simulink model "final_project"  (R2024b)
settings: Solver=FixedStepAuto  StartTime=0.0  StopTime=5  FixedStep=1e-6  RelTol=1e-3
model workspace (MAT data in the model file):
  Vdc = 1200
  fs = 15000
libraries: spsIGBTDiodeLib x6, spsGroundLib x3, simulink x3, spsMultimeterLib x2, spsSeriesRLCBranchLib x2, spsThreePhaseVIMeasurementLib x2, spsAsynchronousMachineSIUnitsLib x1, spsDCVoltageSourceLib x1, spsPower3phInstantaneousLib x1, spsThreePhaseParallelRLCBranchLib x1, spsThreePhaseSeriesRLCBranchLib x1, spsVoltageMeasurementLib x1
settings Model: Creator=zachary.newsom  LastModifiedBy=zachary.newsom

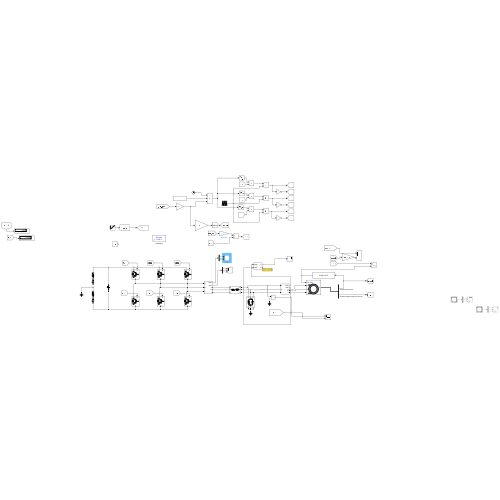
[thumbnail: Simulink's stored preview of the top-level diagram]
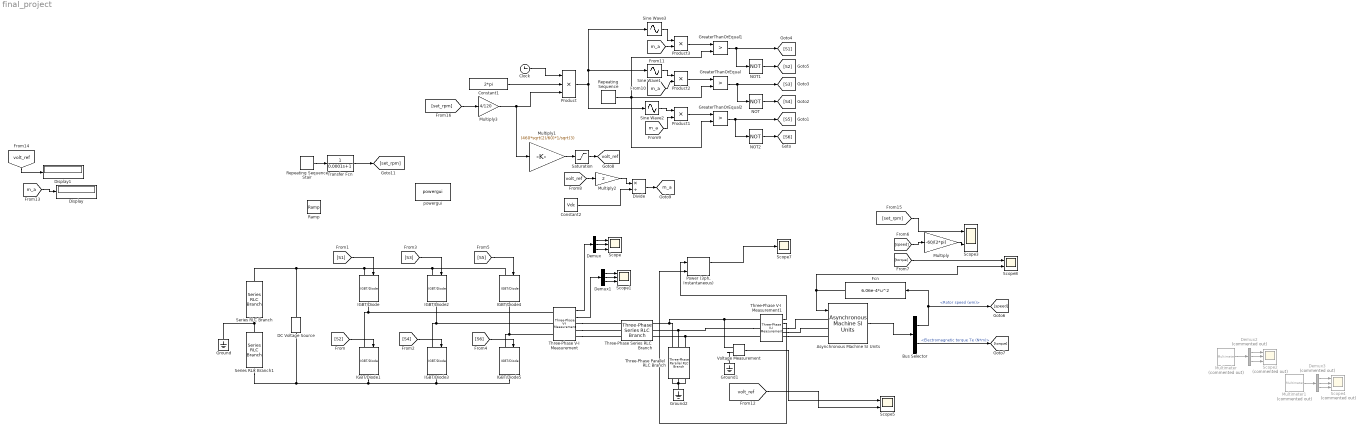
== system final_project ==
  Asynchronous Machine SI Units : spsAsynchronousMachineSIUnitsLib/Asynchronous Machine SI Units  RotorType=Squirrel-cage  PresetModel="01:  5 HP   460 V 60Hz 1750 RPM"  MechanicalLoad=Torque Tm  ShowDetailedParameters=on  ReferenceFrame=Rotor  Units=SI  MeasurementBus=off  NominalParameters=[3730 460 60]  VoltageRatio=1  Stator=[1.115 0.005974]  Rotor=[1.083 0.005974]  Cage1=[0.4155 0.002066]  Cage2=[0.4168 0.0003495]  Lm=0.2037  Mechanical=[0.02 0.005752 2]  PolePairs=2  InitialConditions=[1 0 0 0 0 0 0 0]  SimulateSaturation=off  Saturation=[14.03593122, 27.81365428, 53.79336849, 72.68890987, 97.98006896, 148.6815601, 215.7428561, 302.9841135, 428.7778367 ; 230, 322, 414, 460, 506, 552, 598, 644, 690]  LoadFlowParameters=1492000  TsPowergui=0  TsBlock=-1  IterativeModel=Trapezoidal non iterative  IterativeDiscreteModel=Trapezoidal robust  Pmec=1.492e+006
  Bus Selector : BusSelector  OutputSignals=Mechanical.Rotor speed (wm),Mechanical.Electromagnetic torque Te (N*m)
  Clock : Clock
  Constant1 : Constant  Value=2*pi
  Constant2 : Constant  Value=Vdc
  DC Voltage Source : spsDCVoltageSourceLib/DC Voltage Source  Amplitude=Vdc  Measurements=None
  Demux : Demux  Outputs=3
  Demux1 : Demux  Outputs=3
  Demux2 : Demux  Commented=on  Outputs=3
  Demux3 : Demux  Commented=on  Outputs=3
  Display : Display
  Display1 : Display
  Divide : Product  Inputs=*/
  Fcn : Fcn  Expr=6.06e-4*u^2
  GreaterThanOrEqual : RelationalOperator  Operator=>  OutDataTypeStr=boolean  RndMeth=Simplest  InputSameDT=off
  GreaterThanOrEqual1 : RelationalOperator  Operator=>  OutDataTypeStr=boolean  RndMeth=Simplest  InputSameDT=off
  GreaterThanOrEqual2 : RelationalOperator  Operator=>  OutDataTypeStr=boolean  RndMeth=Simplest  InputSameDT=off
  Ground : spsGroundLib/Ground  LConnTagsString=a
  Ground1 : spsGroundLib/Ground  LConnTagsString=a
  Ground2 : spsGroundLib/Ground  LConnTagsString=a
  IGBT/Diode{,1..3} (4 alike) : spsIGBTDiodeLib/IGBT//Diode  Ron=1e-6  Rs=1e5  Cs=inf  Measurements=off
  IGBT/Diode4 : spsIGBTDiodeLib/IGBT//Diode  Ron=1e-3  Rs=1e5  Cs=inf  Measurements=off
  IGBT/Diode5 : spsIGBTDiodeLib/IGBT//Diode  Ron=1e-3  Rs=1e5  Cs=inf  Measurements=off
  Multimeter : spsMultimeterLib/Multimeter  Commented=on  L=3  sel=1  yselected={}  Gain=0  OutputType=Complex  PlotAtSimulationStop=off  PhasorSimulation=off
  Multimeter1 : spsMultimeterLib/Multimeter  Commented=on  L=3  sel=1  yselected={}  Gain=0  OutputType=Complex  PlotAtSimulationStop=off  PhasorSimulation=off
  Multiply : Gain  Gain=-60/(2*pi)
  Multiply1 : Gain  Gain=(460*sqrt(2)/60)*1/sqrt(3)
  Multiply2 : Gain  Gain=2
  Multiply3 : Gain  Gain=4/120
  NOT : Logic  Operator=NOT  IconShape=distinctive  AllPortsSameDT=off  OutDataTypeStr=boolean
  NOT1 : Logic  Operator=NOT  IconShape=distinctive  AllPortsSameDT=off  OutDataTypeStr=boolean
  NOT2 : Logic  Operator=NOT  IconShape=distinctive  AllPortsSameDT=off  OutDataTypeStr=boolean
  "Power (3ph, Instantaneous)" : spsPower3phInstantaneousLib/Power (3ph, Instantaneous)
  Product : Product  Inputs=3
  Product1 : Product
  Product2 : Product
  Product3 : Product
  Ramp : simulink/Sources/Ramp  slope=1000  start=0  InitialOutput=400
  Repeating Sequence : simulink/Sources/Repeating Sequence  rep_seq_t=[0 0.5 1]/fs  rep_seq_y=[-1 1 -1]
  Repeating Sequence Stair : simulink/Sources/Repeating Sequence Stair  OutValues=[250 500 750 1000 1250 1500 1750].'  tsamp=0.5  OutMin=[]  OutMax=[]  OutDataTypeStr=double  OutputDataTypeScalingMode=double  OutDataType=fixdt(0,8)  ConRadixGroup=Best Precision: Vector-wise  OutScaling=2^-12
  Saturation : Saturate  UpperLimit=Vdc/2  LowerLimit=20
  Scope : Scope  NumInputPorts=3
  Scope1 : Scope  NumInputPorts=3
  Scope2 : Scope  Commented=on  NumInputPorts=3
  Scope3 : Scope  NumInputPorts=2
  Scope4 : Scope  Commented=on  NumInputPorts=3
  Scope5 : Scope  NumInputPorts=2
  Scope7 : Scope
  Scope8 : Scope  NumInputPorts=2
  Series RLC Branch : spsSeriesRLCBranchLib/Series RLC Branch  LConnTagsString=__new0  RConnTagsString=__new0  BranchType=RC  Resistance=1e6  Inductance=1e-3  SetiL0=off  InitialCurrent=0  Capacitance=1e-3  Setx0=off  InitialVoltage=0  Measurements=None
  Series RLC Branch1 : spsSeriesRLCBranchLib/Series RLC Branch  LConnTagsString=__new0  RConnTagsString=__new0  BranchType=RC  Resistance=1e6  Inductance=1e-3  SetiL0=off  InitialCurrent=0  Capacitance=1e-3  Setx0=off  InitialVoltage=0  Measurements=None
  Sine Wave1 : Sin  TimeSource=Use external signal  Phase=2*pi/3  SampleTime=0
  Sine Wave2 : Sin  TimeSource=Use external signal  Phase=4*pi/3  SampleTime=0
  Sine Wave3 : Sin  TimeSource=Use external signal  SampleTime=0
  Three-Phase Parallel RLC Branch : spsThreePhaseParallelRLCBranchLib/Three-Phase Parallel RLC Branch  LConnTagsString=A|B|C  RConnTagsString=A|B|C  BranchType=RC  Resistance=1e6  Inductance=1e-3  Capacitance=258e-6  Measurements=None
  Three-Phase Series RLC Branch : spsThreePhaseSeriesRLCBranchLib/Three-Phase Series RLC Branch  LConnTagsString=A|B|C  RConnTagsString=A|B|C  BranchType=RL  Resistance=0.1  Inductance=2e-3  Capacitance=1e-6  Measurements=Branch currents
  Three-Phase V-I Measurement : spsThreePhaseVIMeasurementLib/Three-Phase V-I Measurement  VoltageMeasurement=phase-to-ground  SetLabelV=off  LabelV=Vabc  Vpu=off  VpuLL=off  CurrentMeasurement=yes  SetLabelI=off  LabelI=Iabc  Ipu=off  Pbase=100e6  Vbase=500e3  OutputType=Complex  PhasorSimulation=off  PSBequivalent=0
  Three-Phase V-I Measurement1 : spsThreePhaseVIMeasurementLib/Three-Phase V-I Measurement  VoltageMeasurement=phase-to-ground  SetLabelV=off  LabelV=Vabc  Vpu=off  VpuLL=off  CurrentMeasurement=yes  SetLabelI=off  LabelI=Iabc  Ipu=off  Pbase=100e6  Vbase=500e3  OutputType=Complex  PhasorSimulation=off  PSBequivalent=0
  Transfer Fcn : TransferFcn  Denominator=[0.0001 1]
  Voltage Measurement : spsVoltageMeasurementLib/Voltage Measurement  PhasorSimulation=off  OutputType=Complex  PSBequivalent=0
  powergui : sps_lib/powergui  Priority=1  SimulationMode=Discrete  SampleTime=1e-6  frequency=60  Iterations=50  frequencyindice=0  Pbase=100e6  ErrMax=1e-4  UnitsV=kV  UnitsW=MW  buscounter=0  FunctionMessages=off  echomessages=off  EnableUseOfTLC=off  CurrentSourceSwitches=off  DisableSnubberDevices=off  DisableRonSwitches=off  DisableVfSwitches=off  DisplayEquations=off  AutomaticDiscreteSolvers=on  SolverType=Tustin/Backward Euler (TBE)  Interpol=off  ExternalGateDelay=off  methode=off  Ts=100  x0status=blocks  SPID=on  SwTol=0  HookPort=off  NonlinearTolerance=1e-6  nMaxIteration=100  ContinueOnMaxIteration=off  RestoreLinks=warning  ResistiveCurrentMeasurement=off  Frange=[0:2:500]  Ylog=off  Xlog=on  ShowGrid=off  save=off  variable=ZData  structure=0  ZoomFFT=off  StartTime=0.0  cycles=1  DisplayStyle=1  fundamental=60  FreqAxis=off  MaxFrequency=1000  frequencyindicesteady=1  RmsSteady=1  display=off
  tag scope: m_a=global, volt_ref=global
  wires:
  [S2] -> IGBT/Diode1/1
  [S1] -> IGBT/Diode/1
  [S4] -> IGBT/Diode3/1
  [S3] -> IGBT/Diode2/1
  [S5] -> IGBT/Diode4/1
  [S6] -> IGBT/Diode5/1
  GreaterThanOrEqual1/1 -> [S1], NOT1/1
  GreaterThanOrEqual2/1 -> [S5], NOT2/1
  GreaterThanOrEqual/1 -> [S3], NOT/1
  Repeating Sequence/1 -> GreaterThanOrEqual1/2, GreaterThanOrEqual/2, GreaterThanOrEqual2/2
  NOT2/1 -> [S6]
  NOT/1 -> [S4]
  NOT1/1 -> [S2]
  Demux/1 -> Scope/1
  Demux/2 -> Scope/2
  Three-Phase V-I Measurement/1 -> Demux/1
  Demux1/3 -> Scope1/3
  Demux1/2 -> Scope1/2
  Demux1/1 -> Scope1/1
  Three-Phase V-I Measurement/2 -> Demux1/1
  Demux2/3 -> Scope2/3
  Demux2/2 -> Scope2/2
  Demux2/1 -> Scope2/1
  Multimeter/1 -> Demux2/1
  Asynchronous Machine SI Units/1 -> Bus Selector/1
  Bus Selector/1 -> [speed], Fcn/1  "<Rotor speed (wm)>"
  Bus Selector/2 -> [torque]  "<Electromagnetic torque Te (N*m)>"
  Demux3/3 -> Scope4/3
  Multimeter1/1 -> Demux3/1
  Demux3/1 -> Scope4/1
  Demux3/2 -> Scope4/2
  Product/1 -> Sine Wave3/1, Sine Wave1/1, Sine Wave2/1
  Constant1/1 -> Product/2
  Sine Wave2/1 -> Product1/1
  Product2/1 -> GreaterThanOrEqual/1
  Sine Wave1/1 -> Product2/1
  Product3/1 -> GreaterThanOrEqual1/1
  Sine Wave3/1 -> Product3/1
  Multiply1/1 -> Saturation/1
  Divide/1 -> [m_a]
  [volt_ref] -> Multiply2/1
  [m_a] -> Product2/2
  [m_a] -> Product1/2
  [m_a] -> Product3/2
  [m_a] -> Display/1
  Three-Phase V-I Measurement1/1 -> "Power (3ph, Instantaneous)"/1
  Three-Phase V-I Measurement1/2 -> "Power (3ph, Instantaneous)"/2
  Multiply2/1 -> Divide/1
  [volt_ref] -> Display1/1
  Voltage Measurement/1 -> Scope5/1
  [volt_ref] -> Scope5/2
  Clock/1 -> Product/1
  [set_rpm] -> Scope3/1
  [torque] -> Scope8/1
  Constant2/1 -> Divide/2
  [speed] -> Multiply/1
  Product1/1 -> GreaterThanOrEqual2/1
  [set_rpm] -> Multiply3/1
  Multiply3/1 -> Product/3, Multiply1/1
  Multiply/1 -> Scope3/2
  Saturation/1 -> [volt_ref]
  Fcn/1 -> Asynchronous Machine SI Units/1, Scope8/2
  Demux/3 -> Scope/3
  "Power (3ph, Instantaneous)"/1 -> Scope7/1
  Repeating Sequence Stair/1 -> Transfer Fcn/1
  Transfer Fcn/1 -> [set_rpm]
  connections:
  IGBT/Diode1/RConn1 -- IGBT/Diode5/RConn1 -- IGBT/Diode3/RConn1 -- Series RLC Branch1/RConn1 -- DC Voltage Source/LConn1
  IGBT/Diode1/LConn1 -- Three-Phase V-I Measurement/LConn1 -- IGBT/Diode/RConn1
  DC Voltage Source/RConn1 -- Series RLC Branch/LConn1 -- IGBT/Diode4/LConn1 -- IGBT/Diode2/LConn1 -- IGBT/Diode/LConn1
  IGBT/Diode3/LConn1 -- IGBT/Diode2/RConn1 -- Three-Phase V-I Measurement/LConn2
  IGBT/Diode5/LConn1 -- IGBT/Diode4/RConn1 -- Three-Phase V-I Measurement/LConn3
  Three-Phase Series RLC Branch/RConn1 -- Three-Phase Parallel RLC Branch/LConn1 -- Voltage Measurement/LConn1 -- Three-Phase V-I Measurement1/LConn1
  Ground2/LConn1 -- Three-Phase Parallel RLC Branch/RConn1 -- Three-Phase Parallel RLC Branch/RConn3 -- Three-Phase Parallel RLC Branch/RConn2
  Ground/LConn1 -- Series RLC Branch1/LConn1 -- Series RLC Branch/RConn1
  Three-Phase V-I Measurement/RConn1 -- Three-Phase Series RLC Branch/LConn1
  Three-Phase V-I Measurement/RConn3 -- Three-Phase Series RLC Branch/LConn3
  Three-Phase V-I Measurement/RConn2 -- Three-Phase Series RLC Branch/LConn2
  Three-Phase V-I Measurement1/LConn2 -- Three-Phase Series RLC Branch/RConn2 -- Three-Phase Parallel RLC Branch/LConn2
  Three-Phase V-I Measurement1/LConn3 -- Three-Phase Series RLC Branch/RConn3 -- Three-Phase Parallel RLC Branch/LConn3
  Three-Phase V-I Measurement1/RConn1 -- Asynchronous Machine SI Units/LConn1
  Three-Phase V-I Measurement1/RConn2 -- Asynchronous Machine SI Units/LConn2
  Three-Phase V-I Measurement1/RConn3 -- Asynchronous Machine SI Units/LConn3
  Voltage Measurement/LConn2 -- Ground1/LConn1
